simulink model "bit32counter"  (R2020a)
settings: Solver=VariableStepAuto  StartTime=0.0  StopTime=10.0  RelTol=1e-3
libraries: simulink_extras x32
settings Model: Creator=kishan  LastModifiedBy=kishan

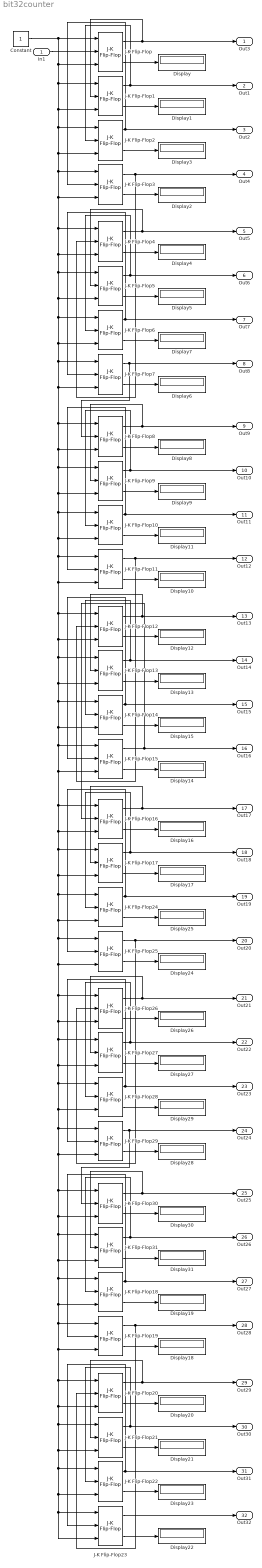
== system bit32counter ==
  In1 : Inport
  Constant : Constant
  Display{,1..31} (32 alike) : Display
  J-K Flip-Flop{,1..31} (32 alike) : simulink_extras/Flip Flops/J-K Flip-Flop  initial_condition=0
  Out3 : Outport
  Out1 : Outport  Port=2
  Out2 : Outport  Port=3
  Out4 : Outport  Port=4
  Out5 : Outport  Port=5
  Out6 : Outport  Port=6
  Out7 : Outport  Port=7
  Out8 : Outport  Port=8
  Out9 : Outport  Port=9
  Out10 : Outport  Port=10
  Out11 : Outport  Port=11
  Out12 : Outport  Port=12
  Out13 : Outport  Port=13
  Out14 : Outport  Port=14
  Out15 : Outport  Port=15
  Out16 : Outport  Port=16
  Out17 : Outport  Port=17
  Out18 : Outport  Port=18
  Out19 : Outport  Port=19
  Out20 : Outport  Port=20
  Out21 : Outport  Port=21
  Out22 : Outport  Port=22
  Out23 : Outport  Port=23
  Out24 : Outport  Port=24
  Out25 : Outport  Port=25
  Out26 : Outport  Port=26
  Out27 : Outport  Port=27
  Out28 : Outport  Port=28
  Out29 : Outport  Port=29
  Out30 : Outport  Port=30
  Out31 : Outport  Port=31
  Out32 : Outport  Port=32
  wires:
  J-K Flip-Flop/1 -> Out3/1, J-K Flip-Flop1/2
  J-K Flip-Flop2/1 -> Out2/1, J-K Flip-Flop3/2
  J-K Flip-Flop1/2 -> Display1/1
  J-K Flip-Flop3/2 -> Display2/1
  J-K Flip-Flop/2 -> Display/1
  J-K Flip-Flop2/2 -> Display3/1
  In1/1 -> J-K Flip-Flop/2
  J-K Flip-Flop1/1 -> Out1/1, J-K Flip-Flop2/2
  J-K Flip-Flop4/1 -> Out5/1, J-K Flip-Flop5/2
  J-K Flip-Flop6/1 -> Out7/1, J-K Flip-Flop7/2
  J-K Flip-Flop5/2 -> Display5/1
  J-K Flip-Flop7/2 -> Display6/1
  J-K Flip-Flop4/2 -> Display4/1
  J-K Flip-Flop6/2 -> Display7/1
  J-K Flip-Flop3/1 -> J-K Flip-Flop4/2, Out4/1
  J-K Flip-Flop5/1 -> Out6/1, J-K Flip-Flop6/2
  J-K Flip-Flop14/1 -> Out15/1, J-K Flip-Flop15/2
  J-K Flip-Flop9/1 -> Out10/1, J-K Flip-Flop10/2
  J-K Flip-Flop7/1 -> J-K Flip-Flop8/2, Out8/1
  J-K Flip-Flop14/2 -> Display15/1
  J-K Flip-Flop8/1 -> Out9/1, J-K Flip-Flop9/2
  J-K Flip-Flop10/1 -> Out11/1, J-K Flip-Flop11/2
  J-K Flip-Flop11/2 -> Display10/1
  J-K Flip-Flop13/1 -> Out14/1, J-K Flip-Flop14/2
  J-K Flip-Flop13/2 -> Display13/1
  J-K Flip-Flop15/2 -> Display14/1
  J-K Flip-Flop8/2 -> Display8/1
  J-K Flip-Flop12/2 -> Display12/1
  J-K Flip-Flop9/2 -> Display9/1
  J-K Flip-Flop12/1 -> Out13/1, J-K Flip-Flop13/2
  J-K Flip-Flop10/2 -> Display11/1
  J-K Flip-Flop11/1 -> J-K Flip-Flop12/2, Out12/1
  J-K Flip-Flop21/1 -> Out30/1, J-K Flip-Flop22/2
  J-K Flip-Flop21/2 -> Display21/1
  J-K Flip-Flop28/1 -> Out23/1, J-K Flip-Flop29/2
  J-K Flip-Flop27/1 -> Out22/1, J-K Flip-Flop28/2
  J-K Flip-Flop29/2 -> Display28/1
  J-K Flip-Flop28/2 -> Display29/1
  J-K Flip-Flop17/1 -> Out18/1, J-K Flip-Flop24/2
  J-K Flip-Flop29/1 -> J-K Flip-Flop30/2, Out24/1
  J-K Flip-Flop25/2 -> Display24/1
  J-K Flip-Flop16/1 -> Out17/1, J-K Flip-Flop17/2
  J-K Flip-Flop22/2 -> Display23/1
  J-K Flip-Flop23/1 -> Out32/1
  J-K Flip-Flop15/1 -> J-K Flip-Flop16/2, Out16/1
  J-K Flip-Flop20/2 -> Display20/1
  J-K Flip-Flop31/2 -> Display31/1
  J-K Flip-Flop27/2 -> Display27/1
  J-K Flip-Flop22/1 -> Out31/1, J-K Flip-Flop23/2
  J-K Flip-Flop26/2 -> Display26/1
  J-K Flip-Flop31/1 -> Out26/1, J-K Flip-Flop18/2
  J-K Flip-Flop20/1 -> Out29/1, J-K Flip-Flop21/2
  J-K Flip-Flop16/2 -> Display16/1
  J-K Flip-Flop18/2 -> Display19/1
  J-K Flip-Flop18/1 -> Out27/1, J-K Flip-Flop19/2
  Constant/1 -> J-K Flip-Flop2/1, J-K Flip-Flop3/1, J-K Flip-Flop6/1, J-K Flip-Flop7/1, J-K Flip-Flop10/1, J-K Flip-Flop11/1, J-K Flip-Flop14/1, J-K Flip-Flop15/1, J-K Flip-Flop24/1, J-K Flip-Flop25/1, J-K Flip-Flop28/1, J-K Flip-Flop29/1, J-K Flip-Flop18/1, J-K Flip-Flop19/1, J-K Flip-Flop22/1, J-K Flip-Flop23/1, J-K Flip-Flop23/3, J-K Flip-Flop22/3, J-K Flip-Flop21/3, J-K Flip-Flop21/1, J-K Flip-Flop20/3, J-K Flip-Flop20/1, J-K Flip-Flop19/3, J-K Flip-Flop18/3, J-K Flip-Flop31/3, J-K Flip-Flop31/1, J-K Flip-Flop30/3, J-K Flip-Flop30/1, J-K Flip-Flop29/3, J-K Flip-Flop28/3, J-K Flip-Flop27/3, J-K Flip-Flop27/1, J-K Flip-Flop26/3, J-K Flip-Flop26/1, J-K Flip-Flop25/3, J-K Flip-Flop24/3, J-K Flip-Flop17/3, J-K Flip-Flop17/1, J-K Flip-Flop16/3, J-K Flip-Flop16/1, J-K Flip-Flop15/3, J-K Flip-Flop14/3, J-K Flip-Flop13/3, J-K Flip-Flop13/1, J-K Flip-Flop12/3, J-K Flip-Flop12/1, J-K Flip-Flop11/3, J-K Flip-Flop10/3, J-K Flip-Flop9/3, J-K Flip-Flop9/1, J-K Flip-Flop8/3, J-K Flip-Flop8/1, J-K Flip-Flop7/3, J-K Flip-Flop6/3, J-K Flip-Flop5/3, J-K Flip-Flop5/1, J-K Flip-Flop4/3, J-K Flip-Flop4/1, J-K Flip-Flop3/3, J-K Flip-Flop2/3, J-K Flip-Flop1/3, J-K Flip-Flop1/1, J-K Flip-Flop/3, J-K Flip-Flop/1
  J-K Flip-Flop24/1 -> Out19/1, J-K Flip-Flop25/2
  J-K Flip-Flop19/1 -> J-K Flip-Flop20/2, Out28/1
  J-K Flip-Flop23/2 -> Display22/1
  J-K Flip-Flop26/1 -> Out21/1, J-K Flip-Flop27/2
  J-K Flip-Flop25/1 -> J-K Flip-Flop26/2, Out20/1
  J-K Flip-Flop24/2 -> Display25/1
  J-K Flip-Flop17/2 -> Display17/1
  J-K Flip-Flop30/1 -> Out25/1, J-K Flip-Flop31/2
  J-K Flip-Flop30/2 -> Display30/1
  J-K Flip-Flop19/2 -> Display18/1
